simulink model "AOT_art"  (R2019b)
settings: Solver=FixedStepAuto  StartTime=0.0  StopTime=10.0  FixedStep=fixedStepSize  RelTol=1e-3
undefined symbols (not defined in the file): artificial_AOT_AFE_max, artificial_AOT_AFE_min, artificial_AOT_ASL_max, artificial_AOT_ASL_min, artificial_AOT_time
settings Model: Creator=JEDDELAN  LastModifiedBy=JEDDELAN
settings DataIOCC: SaveOutput=off  SaveTime=off  ReturnWorkspaceOutputs=off
settings DebuggingCC: ArithmeticOperatorsInVariantConditions=warning
settings SFSimCC: SimUseLocalCustomCode=off  CustomCodeUndefinedFunction=UseInterfaceOnly
settings RTWCC: RTWUseLocalCustomCode=off
settings GRTTargetCC: CombineOutputUpdateFcns=off  MatFileLogging=off

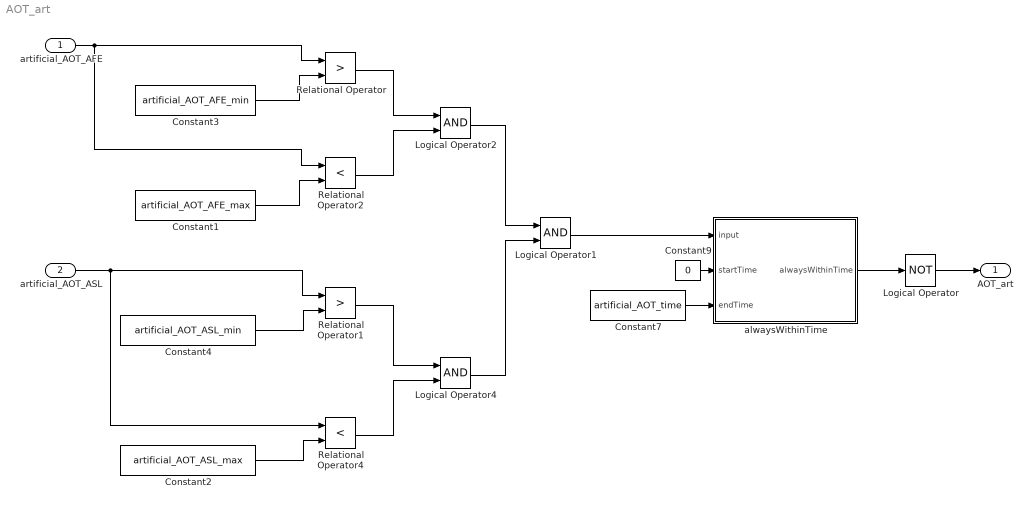
== system AOT_art ==
  artificial_AOT_AFE : Inport
  artificial_AOT_ASL : Inport  Port=2
  Constant1 : Constant  Value=artificial_AOT_AFE_max
  Constant2 : Constant  Value=artificial_AOT_ASL_max
  Constant3 : Constant  Value=artificial_AOT_AFE_min
  Constant4 : Constant  Value=artificial_AOT_ASL_min
  Constant7 : Constant  Value=artificial_AOT_time
  Constant9 : Constant  Value=0
  Logical Operator : Logic  Operator=NOT  AllPortsSameDT=off  OutDataTypeStr=boolean
  Logical Operator1 : Logic  AllPortsSameDT=off  OutDataTypeStr=boolean
  Logical Operator2 : Logic  AllPortsSameDT=off  OutDataTypeStr=boolean
  Logical Operator4 : Logic  AllPortsSameDT=off  OutDataTypeStr=boolean
  Relational Operator : RelationalOperator  Operator=>  OutDataTypeStr=boolean  RndMeth=Simplest
  Relational Operator1 : RelationalOperator  Operator=>  OutDataTypeStr=boolean  RndMeth=Simplest
  Relational Operator2 : RelationalOperator  Operator=<  OutDataTypeStr=boolean  RndMeth=Simplest
  Relational Operator4 : RelationalOperator  Operator=<  OutDataTypeStr=boolean  RndMeth=Simplest
  alwaysWithinTime : Subsystem
      settings: CopyFcn=set_param(gcbh,'LinkStatus','none');
  AOT_art : Outport  OutDataTypeStr=boolean  PortDimensions=1  VectorParamsAs1DForOutWhenUnconnected=off
  wires:
  artificial_AOT_AFE/1 -> Relational Operator2/1, Relational Operator/1
  Relational Operator/1 -> Logical Operator2/1
  Relational Operator2/1 -> Logical Operator2/2
  Constant2/1 -> Relational Operator4/2
  Relational Operator1/1 -> Logical Operator4/1
  Logical Operator2/1 -> Logical Operator1/1
  Constant4/1 -> Relational Operator1/2
  alwaysWithinTime/1(alwaysWithinTime) -> Logical Operator/1
  Constant7/1 -> alwaysWithinTime/3(endTime)
  Constant1/1 -> Relational Operator2/2
  Logical Operator4/1 -> Logical Operator1/2
  Constant9/1 -> alwaysWithinTime/2(startTime)
  artificial_AOT_ASL/1 -> Relational Operator4/1, Relational Operator1/1
  Logical Operator1/1 -> alwaysWithinTime/1(input)
  Relational Operator4/1 -> Logical Operator4/2
  Constant3/1 -> Relational Operator/2
  Logical Operator/1 -> AOT_art/1

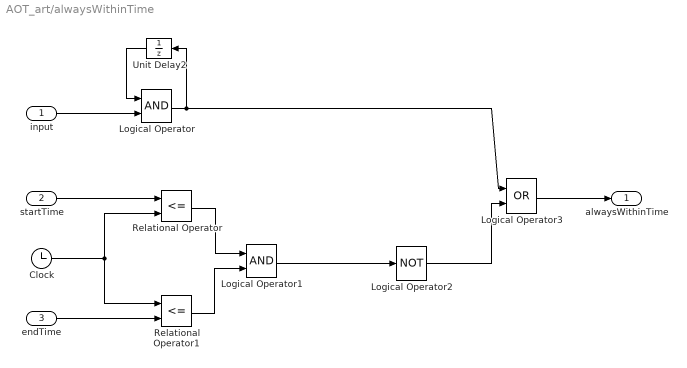
== system AOT_art/alwaysWithinTime ==
  input : Inport
  startTime : Inport  Port=2
  endTime : Inport  Port=3
  Clock : Clock
  Logical Operator : Logic  AllPortsSameDT=off  OutDataTypeStr=boolean
  Logical Operator1 : Logic  AllPortsSameDT=off  OutDataTypeStr=boolean
  Logical Operator2 : Logic  Operator=NOT  AllPortsSameDT=off  OutDataTypeStr=boolean
  Logical Operator3 : Logic  Operator=OR  AllPortsSameDT=off  OutDataTypeStr=boolean
  Relational Operator : RelationalOperator  Operator=<=  OutDataTypeStr=boolean  RndMeth=Simplest
  Relational Operator1 : RelationalOperator  Operator=<=  OutDataTypeStr=boolean  RndMeth=Simplest
  Unit Delay2 : UnitDelay  InitialCondition=1  SampleTime=-1  HasFrameUpgradeWarning=on
  alwaysWithinTime : Outport  VectorParamsAs1DForOutWhenUnconnected=off
  wires:
  startTime/1 -> Relational Operator/1
  Unit Delay2/1 -> Logical Operator/1
  input/1 -> Logical Operator/2
  Logical Operator/1 -> Logical Operator3/1, Unit Delay2/1
  Clock/1 -> Relational Operator1/1, Relational Operator/2
  endTime/1 -> Relational Operator1/2
  Relational Operator1/1 -> Logical Operator1/2
  Relational Operator/1 -> Logical Operator1/1
  Logical Operator1/1 -> Logical Operator2/1
  Logical Operator2/1 -> Logical Operator3/2
  Logical Operator3/1 -> alwaysWithinTime/1
